simulink model "Latest_Greatest_vSandberg"  (R2022b)
settings: Solver=ode4  StartTime=0  StopTime=15  FixedStep=DeltaT  RelTol=1e-6  EnableMultiTasking=on
InitFcn:
  | %run('final_report_initexternal')
  | % Bifocal Relay Mirror Spacecraft (prior to payload installation) Dynamics Simulation          TA Sands
  | clear all;close all;clc;warning off all;
  | 
  | % Simulation run parameters
  | Rate=34.3; Rate=100;  DeltaT=1/Rate;
  | 
  | % Maneuver Parameters
  | roll=0;  pitch=0; yaw=30;   roll=roll*pi/180; pitch=pitch*pi/180; yaw=yaw*pi/180;
  | SlewStart=5; SlewTime=10; SACengage=0;
  | SlewStart=5; SlewTime=5;
  | t0=SlewTime;
  | tf=SlewTime+5;
  | %%
  | 
  | %Constants0
  | Re=6371.2e3;mu=398601.2e9;          %earth radius and universal gravitation constant
  | 
  | % tht=0.5*((sin(pi/SlewTime*(u(4)+2.5)))+1).*[u(1) u(2) u(3)]';
  | % w=(30/77.1239)*0.5*(pi/SlewTime)*((cos(pi/SlewTime*(u(4)+2.5)))+1).*[u(1) u(2) u(3)]'
  | % wdot=-(30/77.1239)*0.5*(pi/SlewTime)^(2)*((sin(pi/SlewTime*(u(4)+2.5)))).*[u(1) u(2) u(3)]'
  | 
  | %compare with differentiating in real time
  | 
  | % A0=[0 0 0];
  | % tht=A0+1/2*(1-cos(pi/SlewTime*(t-SlewStart)))*(A-A0);
  | % w=1/2*(pi/SlewTime)*sin(pi/SlewTime*(t-SlewStart))*(A-A0);
  | % wdot1=1/2*(pi/SlewTime)^2*cos(pi/SlewTime*(t-SlewStart))*(A-A0);
  | 
  | %Spacecraft orbit
  | h=0;                                     %orbit altitude
  | R=Re+h;                             %orbit radius from center of earth
  | we=0.000072921158553;   %earth's angular velocity rad/solar sec(Vallado)
  | wo=sqrt(mu/(Re+h)^3);        %orbit angular velocity
  | incln=36.6001*pi/180;          %Inclination assumed Monterey Latitude
  | epsilon=12*pi/180;  alphao=0;
  | uo=0; nuo=0;                        %Start S/C beneath subsolar point
  | betasun=60; gamma=1.5;
  | a=0.545491852; b=0.314939867;  c=0.704226952;   %Assumed spacecraft rectangular size
  | Area=[b*c a*c a*b];                 %projected area~m^2 in body x,y,z directions
  | density=4.39e-14;
  | kpre=-9.9639/24/3600/180*pi*0;      %nodal precession constant assumed zero here
  | wn=kpre*(Re/(Re+h))^3.5*cos(incln); %nodal precession (zero eccentricity)
  | V=wo*(Re+h);
  | rho=asin(Re/(h+Re));                %earth angular radius
  | Cd=2.5;     psun=4.5E-6;            %Drag coefficient and solar pressure constant~N/m^2
  | Kaero=-0.5*Cd*V^2;   Psolar=2*psun;  %constants for aero and solar torque calculation
  | dL=[0.002 0.002 0.008];             %predicted distance between cp and cg
  | Kme=2.3390e-005;
  | 
  | %Spacecraft Magnetic Properties (assumed)
  | mresid=[0 0 0.01];                  %Spacecraft residual magnetic moment
  | M=mresid;                           %Magnetic unit dipole vector
  | K=7.943e15;
  | 
  | %%
  | % Determining Principal Axes Frame
  | % ACTUAL Spacecraft Inertia conditions
  | Ix=16.67;   Iy=16.67;   Iz=16.67 ;
  | Ixy=0;  Iyz=0;  Ixz=0;
  | Imo=[Ix -Ixy -Ixz;
  |        -Ixy  Iy  -Iyz;
  |        -Ixz -Iyz  Iz];                  %Moment of inertia matrix
  | Iinv=inv(Imo);                      %Moment of inertia inverse goes in dynamics block
  | 
  | % % ACTUAL Spacecraft Inertia conditions
  | Ix=90;   Iy=100;   Iz=250 ;
  | Ixy=-10;  Iyz=20;  Ixz=-10;
  | Imo=[Ix -Ixy -Ixz;
  |        -Ixy  Iy  -Iyz;
  |        -Ixz -Iyz  Iz];                  %Moment of inertia matrix
  | Iinv=inv(Imo);                      %Moment of inertia inverse goes in dynamics block
  | 
  | [p,Ip]=eig(Imo);
  | 
  | %In this case, the principal axes line up with the body axes, otherwise we
  | %would have to examine the principal axes and see which one is closest to
  | %b1, which closest to b2, etc, to determine the order of axis to generate
  | %the DCM
  | bQp=p; %the DCM from principal axis to body are the principal axes we found
  | pQb=bQp.';
  | I1=Ip(1,1);
  | % I1=Imo(1,1);
  | I1inv=1/I1;
  | I2=Ip(2,2);
  | % I2=Imo(2,2);
  | I2inv=1/I2;
  | I3=Ip(3,3);
  | % I3=Imo(3,3);
  | I3inv=1/I3;                    %Moment of inertia inverse goes in dynamics block
  | 
  | 
  | %%
  | %FEEDFORWARD (ASSUMED) Spacecraft Inertia conditions
  | % Ix=119.1259;   Iy=150.6615;   Iz=106.0288;   %ACTUAL Values are Ix=90;   Iy=100;   Iz=250 ;
  | % Ixy=-15.7678;  Iyz=22.31637;  Ixz=-6.54859;  %ACTUAL Values are Ixy=-10;  Iyz=20;  Ixz=-10;
  | % Imo=[Ix -Ixy -Ixz;
  | %        -Ixy  Iy  -Iyz;
  | %        -Ixz -Iyz  Iz];                  %Moment of inertia matrix
  | THETAo=[Ix Ixy Ixz Iy Iyz Iz 0 0 0];
  | theta0=THETAo;
  | % theta0=[0 0 0 0 0 0 0 0 0];
  | %%
  | %Spacecraft initial Euler state angles and rates
  | phio=0;thetao=0;psio=0;                    %Initial Euler Angles
  | phidoto=0;thetadoto=0;psidoto=0;     %Initial Euler Rates
  | 
  | %Calculation of initial quaternion (qo) and angular momentum (Ho)
  | s1=sin(phio/2);s2=sin(thetao/2);s3=sin(psio/2);c1=cos(phio/2);c2=cos(thetao/2);c3=cos(psio/2);
  | q1o=s1*c2*c3-c1*s2*s3;
  | q2o=c1*s2*c3+s1*c2*s3;              %Wie pg. 321
  | q3o=c1*c2*s3-s1*s2*c3;
  | q4o=c1*c2*c3+s1*s2*s3;
  | S1=sin(phio);S2=sin(thetao);S3=sin(psio);C1=cos(phio);C2=cos(thetao);C3=cos(psio);
  | wxo=phidoto-psidoto*S2-wo*S3*C2;
  | wyo=thetadoto*C1+psidoto*C2*S1-wo*(C3*C1+S3*S2*S1);
  | wzo=psidoto*C2*C1-thetadoto*S1-wo*(S3*S2*C1-C3*S1);
  | qo=[q1o q2o q3o q4o];
  | Ho=Imo*[wxo wyo wzo]';
  | norm(Ho)*1000;
  | 
  | %Calculate eclipse time for comparison with EPS calculations
  | Te=100.87*2*V/2/pi;
  | 
  | %CMG Properties (in degrees)
  | %beta=90*pi/180;                                     %Skew angle in degrees converted to radians
  | beta=[90;90;-90;0]; beta=beta.*pi./180;
  | %beta=[54.73;54.73;-54.73;0]; beta=beta.*pi./180;
  | 
  | Gimbal0=[-30*pi/180; 90*pi/180; -30*pi/180;0];   % Initial Gimbal angles for 0 H spin up
  | w_wheel=2800*(2*pi/60);                       %Wheel speed in RPM converted to rad/s
  | Iwheel=0.0614*1.3558179483314;        % Wheel inertia in slug-ft^2 converted (exact) to kg m^2
  | h_wheel=Iwheel*w_wheel;                     % CMG Wheel Angular Momentum
  | 
  | 
  | %I believe Smeresky Rizzo did
  | %     PID_case = 1;  % Feedback controller method 1=PDI, 2=Matlab PID
  | %     kp = 1000;  % Kp gain for controller
  | %     kd = 10;  % Kd gain for controller
  | %     ki = 0.1;  % Ki gain for controller
  | %
  | %     observer_case = 2;  % 1 = observer off, 2 = observer on
  | %     kp2 = 1000;  % Kp gain for controller
  | %     kd2 = 10;  % Kd gain for controller
  | %     ki2 = 0.1;  % Ki gain for controller
  | %and used enhance PDI not just PD
  | 
  | %Smeresky Rizzo also uses
  | % J = [2.0 .1 .1; .1 2.0 .1; .1 .1 2.0]; %For an uglier J at the start time
  | % J2 = J*.2;
  | 
  | % [Fossen]'s adaptive feedforward parameters
  | ETA=1;LAMBDA=10;  uffGain=1;
  | ETA=30;
  | gamma_ff=30;
  | lambda_r=1/2; %lambda for calculation of the reference trajectories
  | lambda_r=100;
  | 
  | %FEEDBACK CONTROLLERS Follow
  | %PDI Controller Gains  % TUNED Well for Presence of LOWPASS (Kp=0.5; Kd=Kp*750;  Ki=0.1)
  | %Kp=0.5;  Kd=Kp*750;  Ki=0.1;
  | 
  | %PDI Controller Gains  % TUNED WELL FOR NO-NOISE (Kp=1; Kd=2000*Kp; Ki=5)
  | Kp=1;   Kd=Kp*6000;    Ki=5;
  | Kp=1;   Kd=1000;    Ki=1;
  | 
  | %gains for Slotine Ex 9.5
  | Kd=200;
  | Kp=Kd*lambda_r;
  | % Kp=2000;
  | 
  | %gains for Improved Hamiltonian Control
  | Kp=100;
  | Kd=200;
  | 
  | %gains for Smeresky Rizzo
  | Kp=1000*100;
  | Kd=10*100;
  | Ki=0.1*100; %added the 100 because their Inertia was about 100 times smaller
  | 
  | Ki=0;
  | 
  | %PDI Controller Gains  % TUNED WELL FOR NOISE (Kp=1; Kd=Kp*3000; Ki=1)
  | %Kp=1;   %Kd=Kp*3000;   %Ki=1;
  | 
  | %PID Controller Gains tuned well for uff and ufb decoupling
  | Kpx=1;  Kdx=1000;  Kix=-1;
  | Kpx=20;  Kdx=1000;  Kix=0.1;N_pid=100;
  | %Kpx=16.9;  Kdx=87.58;  Kix=0.8009; N_pid=5.454;
  | %Kpx=19.61;  Kdx=258.9;  Kix=0.3299; N_pid=329.6;
  | Kpx=233.9;  Kdx=890.9;  Kix=13.64; N_pid=1143;
  | Kpx=20;  Kdx=1000;  Kix=0.1;N_pid=100;
  | Kpx=100000;Kix=0.1*100;
  | %Bandpass filter pole per Bong Wie 2nd Edition pg 137-138
  | wp=10*pi/SlewTime;       % Product of pole frequency and zero frequency establishes max phase lag
  | wz=2*wp;
  | dampZ=1;  % >0 but small for good tracking..
  | dampP=dampZ;
  | % Sensor Noise Parameters
  | NoiseVariance=1e-9;             BADNoiseVariance=NoiseVariance*1e3;
  | 
  | % Observer Gains
  | MaxI=300;  lambda1=12.5  ;   lambda2=50 ;   lambda3= 200;
  | Kdo=MaxI*(lambda1+lambda2+lambda3)/10;
  | Kpo=MaxI*(lambda1*(lambda2+lambda3)+lambda2*lambda3)/10;
  | Kio=MaxI*lambda1*lambda2*lambda3/9;
  | 
  | % Kdo=1;Kpo=1;Kio=1;
  | Kdo=100;
  | Kpo=1000;
  | Kio=1000;
  | 
  | m=100*eye(3);
  | minv=pinv(m);
  | m=100;
  | x0=[R;0;0];
  | xdot0= cross([0;0;wo], x0);
  | m=100;
  | mi=1/m;
  | 
  | % Working on different parameterizations
  | % making all parameterizations the same size as the 9 parameterization,
  | % by omitting some values
  | % [u(4) 0 0 -u(2)*u(3) 0 u(3)*u(2) 0 0 0;u(1)*u(3) 0 0 u(5) 0 -u(3)*u(1) 0 0 0;-u(1)*u(2) 0 0 u(2)*u(1) 0 u(6) 0 0 0]
  | % [u(4) u(5) u(6) -u(2)*u(3) 0 u(3)*u(2) 0 0 0;u(1)*u(3) u(4) 0 u(5) u(6) -u(3)*u(1) 0 0 0;-u(1)*u(2) 0 u(4) u(2)*u(1) u(5) u(6) 0 0 0]
  | %make sure to look at what exactly theta0 is
  | 
  | 
  | 
  | % z=[u(1);u(2);u(3)]+([u(4);u(5);u(6)]-[u(1);u(2);u(3)])/2*(1+sin(pi/SlewTime*(u(8)+3*SlewTime/2-u(7))))
  | %
  | % zdot=([u(4);u(5);u(6)]-[u(1);u(2);u(3)])/2*(pi/SlewTime)*(cos(pi/SlewTime*(u(8)+3*SlewTime/2-u(7))))
  | %
  | % zddot=-([u(4);u(5);u(6)]-[u(1);u(2);u(3)])/2*(pi/SlewTime)^2*(sin(pi/SlewTime*(u(8)+3*SlewTime/2-u(7))))
  | 
  | tic
StopFcn:
  | toc
  | %run('final_report_stopexternal')
  | 
  | if flag==0; Hcmg=Hcmg;else;Hcmg=HcmgMP;end;
  | Hxcmg=[];Hycmg=[];Hzcmg=[];CondA=[]; CondA_MP=[];t=[]; SingPt=[];DetA=[];
  | for i=1:max(size(A));  t=[t i*DeltaT];  H=Hcmg(:,:,i); Hx=H(1,:);  Hy=H(2,:);  Hz=H(3,:);
  | detA=det(A(:,1:3,i));Hxcmg=[Hxcmg Hx];  Hycmg=[Hycmg Hy];  Hzcmg=[Hzcmg Hz];
  | CONDA=cond(A(:,:,i));
  | DetA=[DetA detA]; DetA=1./DetA;
  | CondA=[CondA CONDA];end;   %CondA=CondA./max(CondA); DetA=DetA./max(DetA);
  | Hmag=sqrt(Hxcmg.^2+Hycmg.^2+Hzcmg.^2);x=(max(t)-DeltaT);
  | 
  | InvCondA;
  | 
  | if flag==0; MaxInvCond=min(1./CondA(10*Rate+1:end));DELTA=delta;DELTAdot=deltadot;
  | else; MaxInvCond=min(1./CondA_MP(10*Rate+1:end));DELTA=delta_MP;DELTAdot=deltadot_MP;Hcmg=HcmgMP;end;
  | %
  | ERROR=(trajectory*180/pi-Euler);
  | 
  | figure(1); wdotTrajectory=[CMDTrajectory(:,1) CMDTrajectory(:,2) CMDTrajectory(:,3)];  wTrajectory=[CMDTrajectory(:,4) CMDTrajectory(:,5) CMDTrajectory(:,6)]; ThetaTrajectory=180/pi.*[trajectory(:,1) trajectory(:,2) trajectory(:,3)]; set(gca,'fontsize',32, 'fontname','Palatino Linotype');
  | subplot(3,1,1); plot(t,wdotTrajectory, 'linewidth',2); axis tight; grid; ylabel('\omega^d^o^t_C_M_D (deg)','fontsize',32); title('Desired Angle, Rate, Acceleration Trajectories','fontsize',32);   set(gca,'XTick',0:2:15);     set(gca,'XTickLabel',{' ',' ',' ',' ',' ',' ',' ',' ','15'}); set(gca,'fontsize',32, 'fontname','Palatino Linotype');
  | subplot(3,1,2); plot(t,wTrajectory,'linewidth',2); axis tight; grid; ylabel('\omega_C_M_D (deg)','fontsize',32);set(gca,'XTick',0:2:15);     set(gca,'XTickLabel',{' ',' ',' ',' ',' ',' ',' ',' ','15'}); set(gca,'fontsize',32, 'fontname','Palatino Linotype');
  | subplot(3,1,3); plot(t,ThetaTrajectory,'linewidth',2); axis tight; grid; ylabel('\theta_C_M_D (deg)','fontsize',32); xlabel('time (sec)','fontsize',32); set(gca,'fontsize',32, 'fontname','Palatino Linotype');
  | 
  | % figure(2);
  | % subplot(2,1,1);plot(t,Hmag,'LineWidth',3);   ylabel('|H_c_m_g|','Fontsize',16);grid;axis([0,x,0,3]); set(gca,'fontsize',16);set(gca,'XTickLabel',{' ',' ',' ',' ',' ',' ',' ',' ','15'});
  | % subplot(2,1,2);plot(t,InvCondA,'linewidth',3);grid;xlabel('t(sec)','fontsize',14,'fontname','times');ylabel('Cond[A]','fontsize',14,'fontname','times');axis([0,max(t),0,21.82]); set(gca,'fontsize',16);
  | %
  | % DELTA1=DELTA(1,:);DELTA2=DELTA(2,:);DELTA3=DELTA(3,:);DELTA4=DELTA(4,:);
  | % DELTAdot1=DELTAdot(1,:);DELTAdot2=DELTAdot(2,:);DELTAdot3=DELTAdot(3,:);DELTAdot4=DELTAdot(4,:);
  | %
  | % figure(3);subplot(4,1,1);plot(t,DELTA1,'LineWidth',3); title('Gimbal Angles','fontsize',16);ylabel('\theta_1(deg)','Fontsize',14);grid;axis tight; set(gca,'XTickLabel',{' ',' ',' ',' ',' ',' ',' ',' ','15'});set(gca,'fontsize',16);
  | % subplot(4,1,2);plot(t,DELTA2,'LineWidth',3); ylabel('\theta_2(deg)','Fontsize',16);grid;axis tight; set(gca,'XTickLabel',{' ',' ',' ',' ',' ',' ',' ',' ','15'});set(gca,'fontsize',16);
  | % subplot(4,1,3);plot(t,DELTA3,'LineWidth',3); ylabel('\theta_3(deg)','Fontsize',16);grid;axis tight; set(gca,'XTickLabel',{' ',' ',' ',' ',' ',' ',' ',' ','15'});set(gca,'fontsize',16);
  | % subplot(4,1,4);plot(t,InvCondA,'linewidth',3);grid;xlabel('t(sec)','fontsize',14,'fontname','times');ylabel('Cond[A]','fontsize',14,'fontname','times');axis([0,max(t),0,21.82]); set(gca,'fontsize',16);
  | %
  | % figure(4);subplot(4,1,1);plot(t,DELTAdot1,'LineWidth',3);  title('Gimbal Angle RATES','fontsize',16); ylabel('\theta_d_o_t_1(rad/s)','Fontsize',16);grid; axis([0,x,-pi*1.1,pi*1.1]);   set(gca,'XTickLabel',{' ',' ',' ',' ',' ',' ',' ',' ','15'});set(gca,'fontsize',16);
  | % subplot(4,1,2);plot(t,DELTAdot2,'LineWidth',3);   ylabel('\theta_d_o_t_2(rad/s)','Fontsize',16);grid;axis([0,x,-pi*1.1,pi*1.1]);   set(gca,'XTickLabel',{' ',' ',' ',' ',' ',' ',' ',' ','15'});   set(gca,'fontsize',16);
  | % subplot(4,1,3);plot(t,DELTAdot3,'LineWidth',3);   ylabel('\theta_d_o_t_3(rad/s)','Fontsize',16);grid;axis([0,x,-pi*1.1,pi*1.1]); set(gca,'XTickLabel',{' ',' ',' ',' ',' ',' ',' ',' ','15'});set(gca,'fontsize',16);
  | % subplot(4,1,4);plot(t,InvCondA,'linewidth',3);grid;xlabel('t(sec)','fontsize',14,'fontname','times');ylabel('Cond[A]','fontsize',14,'fontname','times');axis([0,max(t),0,21.82]); set(gca,'fontsize',16);
  | %
  | % figure(5);
  | % subplot(4,1,1);plot(t,Hxcmg,'linewidth',3);axis([0,x,-3.25,3.25]);grid;ylabel('h_x/|h|','fontsize',16);title('Normalized Momentum','fontsize',16);set(gca,'XTickLabel',{' ',' ',' ',' ',' ',' ',' ',' ','15'});set(gca,'fontsize',16);
  | % subplot(4,1,2);plot(t,Hycmg,'linewidth',3);axis([0,x,-3.25,3.25]);grid;ylabel('h_y/|h|','fontsize',16);set(gca,'XTickLabel',{' ',' ',' ',' ',' ',' ',' ',' ','15'});set(gca,'fontsize',16);
  | % subplot(4,1,3);plot(t,Hzcmg,'linewidth',3);axis([0,x,-3.25,3.25]);grid;ylabel('h_z/|h|','fontsize',16);  set(gca,'XTickLabel',{' ',' ',' ',' ',' ',' ',' ',' ','15'});set(gca,'fontsize',16);
  | % subplot(4,1,4);plot(t,InvCondA,'linewidth',3);grid;xlabel('t(sec)','fontsize',14,'fontname','times');ylabel('Cond[A]','fontsize',14,'fontname','times');axis([0,max(t),0,21.82]); set(gca,'fontsize',16);
  | %
  | figure(6); EulerX=Euler(:,1);EulerY=Euler(:,2);EulerZ=Euler(:,3);
  | subplot(4,1,1);plot(t,EulerX,'linewidth',3); axis([0,x,min(EulerX),max(EulerX)]);grid;ylabel('\phi(deg)','fontsize',32);title('True Euler Angles','fontsize',14);  set(gca,'XTickLabel',{' ',' ',' ',' ',' ',' ',' ',' ','15'});  set(gca,'fontsize',32, 'fontname','Palatino Linotype');
  | subplot(4,1,2);plot(t,EulerY,'linewidth',3);  axis([0,x,min(EulerY),max(EulerY)]); grid;ylabel('\theta(deg)','fontsize',32);  set(gca,'XTickLabel',{' ',' ',' ',' ',' ',' ',' ',' ','15'}); set(gca,'fontsize',32, 'fontname','Palatino Linotype');
  | subplot(4,1,3);plot(t,EulerZ,'linewidth',3);axis([0,x,min(EulerZ),max(EulerZ)]);grid;  ylabel('\psi(deg)','fontsize',32);  set(gca,'XTickLabel',{' ',' ',' ',' ',' ',' ',' ',' ','15'});  set(gca,'fontsize',32, 'fontname','Palatino Linotype');
  | subplot(4,1,4);plot(t,InvCondA,'linewidth',3);grid;xlabel('t(sec)','fontsize',32,'fontname','times');ylabel('Cond[A]','fontsize',14,'fontname','times');axis([0,max(t),0,21.82]); set(gca,'fontsize',32, 'fontname','Palatino Linotype');
  | 
  | EX=ERROR(:,1);  EY=ERROR(:,2);     EZ=ERROR(:,3);
  | MeanXerror=mean(EX); Xmean=num2str(MeanXerror); xmean=['\mu_\phi=', Xmean];
  | STDx=std(EX);Xsigma=num2str(STDx);SigmaX=['    \sigma_x=' Xsigma];  xlegend=[xmean, SigmaX];
  | MeanYerror=mean(EY); Ymean=num2str(MeanYerror); ymean=['\mu_\theta=', Ymean];
  | STDy=std(EY); Ysigma=num2str(STDy);SigmaY=['    \sigma_y=' Ysigma]; ylegend=[ymean, SigmaY];
  | MeanZerror=mean(EZ); Zmean=num2str(MeanZerror); zmean=['\mu_\psi=', Zmean];
  | STDz=std(EZ);Zsigma=num2str(STDz);SigmaZ=['    \sigma_z=' Zsigma]; zlegend=[zmean, SigmaZ];
  | MeanError=[MeanXerror MeanYerror MeanZerror];  StdDev=[STDx STDy STDz];
  | 
  | figure(7);
  | subplot(3,1,1);plot(t,EX,'linewidth',3);    axis([0,x,min(EX)*1.25,max(EX)*1.25]);  title('Euler Angle Tracking Error','fontsize',16); set(gca,'fontsize',32, 'fontname','Palatino Linotype');
  |      legend(xlegend, 'location','NorthEast');  grid   ; ylabel('\phi(deg)','fontsize',32);set(gca,'XTickLabel',{' ',' ',' ',' ',' ',' ',' ',' ','15'}); set(gca,'fontsize',32, 'fontname','Palatino Linotype');
  | subplot(3,1,2);plot(t,EY,'linewidth',3);   axis([0,x,min(EY)*1.25,max(EY)*1.25]);
  |       legend(ylegend, 'location','NorthEast');  grid;    ylabel('\theta(deg)','fontsize',32);set(gca,'XTickLabel',{' ',' ',' ',' ',' ',' ',' ',' ','15'}); set(gca,'fontsize',32, 'fontname','Palatino Linotype');
  | subplot(3,1,3);plot(t,EZ,'linewidth',3);    axis([0,x,min(EZ)*1.25,max(EZ)*1.25]);
  |      legend(zlegend, 'location','NorthEast');  grid;   ylabel('\psi(deg)','fontsize',32);xlabel('t(sec)','fontsize',16); set(gca,'fontsize',32, 'fontname','Palatino Linotype');
  | %
  | % figure(8);subplot(3,3,1);
  | % plot(t,THETAhat(:,1),'linewidth',2);grid; axis tight;ylabel('J_x_x','fontsize',16);  set(gca,'XTickLabel',{' ',' ',' ',' ',' ',' ',' ',' ','15'});  set(gca,'fontsize',16);
  | % subplot(3,3,2);plot(t,THETAhat(:,2),'linewidth',3);grid;axis tight;ylabel('J_x_y','fontsize',16);   set(gca,'XTickLabel',{' ',' ',' ',' ',' ',' ',' ',' ','15'});  set(gca,'fontsize',16);  title('Inertia & Momentum Adaption','fontsize',18);
  | % subplot(3,3,3);plot(t,THETAhat(:,3),'linewidth',3);grid;axis tight;ylabel('J_x_z','fontsize',16);set(gca,'XTickLabel',{' ',' ',' ',' ',' ',' ',' ',' ','15'});set(gca,'fontsize',16);
  | % subplot(3,3,4);plot(t,THETAhat(:,4),'linewidth',3);grid;axis tight;ylabel('J_y_y','fontsize',16);set(gca,'XTickLabel',{' ',' ',' ',' ',' ',' ',' ',' ','15'});set(gca,'fontsize',16);
  | % subplot(3,3,5);plot(t,THETAhat(:,5),'linewidth',3);grid;axis tight;ylabel('J_y_z','fontsize',16);set(gca,'XTickLabel',{' ',' ',' ',' ',' ',' ',' ',' ','15'});set(gca,'fontsize',16);
  | % subplot(3,3,6);plot(t,THETAhat(:,6),'linewidth',3);grid;axis tight;ylabel('J_z_z','fontsize',16);set(gca,'XTickLabel',{' ',' ',' ',' ',' ',' ',' ',' ','15'});set(gca,'fontsize',16);
  | % subplot(3,3,7);plot(t,THETAhat(:,7),'linewidth',3);grid;axis tight;ylabel('H_x','fontsize',16);xlabel('t(sec)','fontsize',14);set(gca,'fontsize',16);
  | % subplot(3,3,8);plot(t,THETAhat(:,8),'linewidth',3);grid;axis tight;ylabel('H_y','fontsize',16);xlabel('t(sec)','fontsize',14);set(gca,'fontsize',16);
  | % subplot(3,3,9);plot(t,THETAhat(:,9),'linewidth',3);grid;axis tight;ylabel('H_z','fontsize',16);xlabel('t(sec)','fontsize',14);set(gca,'fontsize',16);
  | %
  | ControlX=sqrt(abs(ControlEffort(end,1)))/(max(t)); ControlStringX=num2str(ControlX); Control_x=['1/t sqrt(\int u^2_\phi dt)=', ControlStringX];
  | ControlY=sqrt(abs(ControlEffort(end,2)))/(max(t)); ControlStringY=num2str(ControlY); Control_y=['1/t sqrt(\int u^2_\theta dt)=', ControlStringY];
  | ControlZ=sqrt(abs(ControlEffort(end,3)))/(max(t)); ControlStringZ=num2str(ControlZ); Control_z=['1/t sqrt(\int u^2_\psi dt)=', ControlStringZ];
  | 
  | figure(9);
  | subplot(2,1,1);plot(t,ufb,'linewidth',3);grid; axis tight;ylabel('Feedback Control (Nm)','fontname','times','fontsize',32);  legend(Control_x, Control_y, Control_z, 'location','SouthEast'); set(gca,'fontsize',32, 'fontname','Palatino Linotype');
  | title('Feedforward and Feedback Controls','fontsize',18);set(gca,'XTickLabel',{' ',' ',' ',' ',' ',' ',' ',' ','15'}); set(gca,'fontsize',32, 'fontname','Palatino Linotype');
  | subplot(2,1,2);plot(t,uff,'linewidth',3);grid; axis tight; ylabel('FeedForward Control (Nm)','fontname','times','fontsize',32);      xlabel('time(sec)','fontname','times','fontsize',14); set(gca,'fontsize',32, 'fontname','Palatino Linotype');
  | 
  | figure(10);
  | subplot(4,1,1);plot(t,ufb(:,1),'linewidth',3);grid;ylabel('u_\phi(Nm)','fontsize',32);title('u_f_b (Nm)','fontsize',32); axis tight; set(gca,'XTickLabel',{' ',' ',' ',' ',' ',' ',' ',' ','15'});set(gca,'fontsize',32, 'fontname','Palatino Linotype');
  | subplot(4,1,2);plot(t,ufb(:,2),'linewidth',3); grid;ylabel('u_\theta(Nm)','fontsize',32); axis tight; set(gca,'XTickLabel',{' ',' ',' ',' ',' ',' ',' ',' ','15'}); set(gca,'fontsize',32, 'fontname','Palatino Linotype');
  | subplot(4,1,3);plot(t,ufb(:,3),'linewidth',3); grid;ylabel('u_\psi(Nm)','fontsize',32); axis tight; set(gca,'XTickLabel',{' ',' ',' ',' ',' ',' ',' ',' ','15'}); set(gca,'fontsize',32, 'fontname','Palatino Linotype');
  | subplot(4,1,4);plot(t,InvCondA,'linewidth',3);grid;xlabel('t(sec)','fontsize',32,'fontname','times');ylabel('Cond[A]','fontsize',32,'fontname','times');axis([0,max(t),0,21.82]); set(gca,'fontsize',32, 'fontname','Palatino Linotype');
  | 
  | % % CALCULATE FIGURES OF MERIT FOR ESTIMATION ACCURACY OF LUENBERGER OBSERVER
  | % EEX=EstimationError(:,1);EEY=EstimationError(:,2);EEZ=EstimationError(:,3);
  | % MeanEEX=mean(EEX); EEXmean=num2str(MeanEEX); Exmean=['Luenberger \mu_\phi^o _E_r_r_o_r=', EEXmean];
  | % MeanEEY=mean(EEY); EEYmean=num2str(MeanEEY); Eymean=['Luenberger \mu_\theta^o _E_r_r_o_r=', EEYmean];
  | % MeanEEZ=mean(EEZ); EEZmean=num2str(MeanEEZ); Ezmean=['Luenberger \mu_\psi^o _E_r_r_o_r=', EEZmean];
  | % STDEEX=std(EEX);                      EEXstd=num2str(STDEEX);         Exstd=['   \sigma_\phi^o _E_r_r_o_r=', EEXstd];
  | % STDEEY=std(EEY);                      EEYstd=num2str(STDEEY);         Eystd=['   \sigma_\theta^o _E_r_r_o_r=', EEYstd];
  | % STDEEZ=std(EEZ);                      EEZstd=num2str(STDEEZ);         Ezstd=['   \sigma_\psi^o _E_r_r_o_r=', EEZstd];
  | % XlabelLuen=[Exmean Exstd];  YlabelLuen=[Eymean Eystd];  ZlabelLuen=[Ezmean Ezstd];
  | %
  | % % CALCULATE FIGURES OF MERIT FOR ESTIMATION ACCURACY OF PID OBSERVERS
  | % EEXo=PIDoEstimationError(:,1);EEYo=PIDoEstimationError(:,2);EEZo=PIDoEstimationError(:,3);
  | % MeanEEXo=mean(EEXo); EEXmeano=num2str(MeanEEXo); Exmeano=['PID \mu_\phi^o _E_r_r_o_r=', EEXmeano];
  | % MeanEEYo=mean(EEYo); EEYmeano=num2str(MeanEEYo); Eymeano=['PID \mu_\theta^o _E_r_r_o_r=', EEYmeano];
  | % MeanEEZo=mean(EEZo); EEZmeano=num2str(MeanEEZo); Ezmeano=['PID \mu_\psi^o _E_r_r_o_r=', EEZmeano];
  | % STDEEXo=std(EEXo);                      EEXstdo=num2str(STDEEXo);         Exstdo=['    \sigma_\phi^o _E_r_r_o_r=', EEXstdo];
  | % STDEEYo=std(EEYo);                      EEYstdo=num2str(STDEEYo);         Eystdo=['    \sigma_\theta^o _E_r_r_o_r=', EEYstdo];
  | % STDEEZo=std(EEZo);                      EEZstdo=num2str(STDEEZo);         Ezstdo=['    \sigma_\psi^o _E_r_r_o_r=', EEZstdo];
  | % XlabelPID=[Exmeano Exstdo];  YlabelPID=[Eymeano Eystdo];  ZlabelPID=[Ezmeano Ezstdo];
  | %
  | % % CALCULATE FIGURES OF MERIT FOR ESTIMATION ACCURACY OF KALMAN OBSERVERS
  | % EEXkf=KalmanEstimationError(:,1);   EEYkf=KalmanEstimationError(:,2);        EEZkf=KalmanEstimationError(:,3);
  | % MeanEEXkf=mean(EEXkf);                EEXmeankf=num2str(MeanEEXkf);         Exmeankf=['Kalman \mu_\phi^o _E_r_r_o_r=', EEXmeankf];
  | % MeanEEYkf=mean(EEYkf);                EEYmeankf=num2str(MeanEEYkf);         Eymeankf=['Kalman \mu_\theta^o _E_r_r_o_r=', EEYmeankf];
  | % MeanEEZkf=mean(EEZkf);                EEZmeankf=num2str(MeanEEZkf);         Ezmeankf=['Kalman \mu_\psi^o _E_r_r_o_r=', EEZmeankf];
  | % STDEEXkf=std(EEXkf);                      EEXstdkf=num2str(STDEEXkf);         Exstdkf=['    \sigma_\phi^o _E_r_r_o_r=', EEXstdkf];
  | % STDEEYkf=std(EEYkf);                      EEYstdkf=num2str(STDEEYkf);         Eystdkf=['    \sigma_\theta^o _E_r_r_o_r=', EEYstdkf];
  | % STDEEZkf=std(EEZkf);                      EEZstdkf=num2str(STDEEZkf);         Ezstdkf=['    \sigma_\psi^o _E_r_r_o_r=', EEZstdkf];
  | % Xlabelkf=[Exmeankf Exstdkf];  Ylabelkf=[Eymeankf Eystdkf];  Zlabelkf=[Ezmeankf Ezstdkf];
  | %
  | %figure(11);
  | %subplot(3,1,1);plot(t,KalmanEstimationError(:,1),'r:','linewidth',3); hold on; plot(t,PIDoEstimationError(:,1),'linewidth',3);  plot(t,EstimationError(:,1),'k--','linewidth',3);   set(gca,'fontsize',12);
  | %ylabel('\phi Roll (deg)','fontsize',16);   title('Observer Estimation Error Comparison','fontsize',14);  legend(Xlabelkf,XlabelPID, XlabelLuen, 'location','NorthWest'); grid; axis([0,15,-0.01,0.04]);
  | %set(gca,'XTickLabel',{' ',' ',' ',' ',' ',' ',' ',' ','15'});
  | 
  | %subplot(3,1,2); plot(t,KalmanEstimationError(:,2),'r:','linewidth',3); hold on;  plot(t,PIDoEstimationError(:,2),'linewidth',3); plot(t,EstimationError(:,2),'k--','linewidth',3); set(gca,'fontsize',12);
  | %ylabel('\theta Pitch (deg)','fontsize',16); hold off;  legend(Ylabelkf, YlabelPID, YlabelLuen, 'location','SouthWest'); grid;  set(gca,'XTickLabel',{' ',' ',' ',' ',' ',' ',' ',' ','15'});  axis([0,15,-0.08,0.03]);
  | 
  | %subplot(3,1,3); plot(t,KalmanEstimationError(:,3),'r:','linewidth',3);  hold on;  plot(t,PIDoEstimationError(:,3),'linewidth',3);plot(t,EstimationError(:,3),'k--','linewidth',3);set(gca,'fontsize',12);
  | %ylabel('\psi Yaw (deg)','fontsize',16);xlabel('t(sec)','fontsize',16);  hold off;  legend(Zlabelkf, ZlabelPID, ZlabelLuen,'location','NorthWest'); grid; axis tight;
  | 
  | %openfig('90_Degree_Singularity_Hypersurface');hold on;plot3(Hcmg(1,:),Hcmg(2,:),Hcmg(3,:), 'LineWidth',3);hold off;
  | 
  | 
  | 
  | figure(12)
  | plot(t,EX*pi/180,'linewidth',2)
  | hold on
  | plot(t,EY*pi/180,'linewidth',2)
  | plot(t,EZ*pi/180,'linewidth',2)
  | hold off
  | grid;
  | set(gca,'fontsize',32, 'fontname','Palatino Linotype');
  | %
  | % figure(13)
  | % plot(t,Euler(:,1)-30,'linewidth',2)
  | 
  | 
  | figure(13)
  | plot(t,Euler(:,1),'linewidth',2); hold on
  | plot(t,Euler(:,2),'linewidth',2); plot(t,Euler(:,3),'linewidth',2); hold off
  | cost=[' J=' num2str(sum(ControlEffort(end,:))) ';'];
  | time=[' RunTime=' num2str(toc) ';'];
  | theta_final=[' \theta(t_f)= ' num2str(Euler(end,1)) ';' cost time];
  | phi_final=[' \phi(t_f)= ' num2str(Euler(end,2)) ';'];
  | psi_final=[' \psi(t_f)= ' num2str(Euler(end,3)-30) ';'];
  | legend(theta_final,phi_final,psi_final); grid;
  | set(gca,'fontsize',32, 'fontname','Palatino Linotype');
  | 
  | % figure; grid on;
  | % plot3(r(:,1),r(:,2),r(:,3),'Linewidth',1.5);
  | %
  | % figure; grid on;
  | % plot3(r1(:,1),r1(:,2),r1(:,3),'Linewidth',1.5);
  | %
  | % plot(t,quat_error)
  | % set(gca,'fontsize',20)
undefined symbols (not defined in the file): magnitude, svd
libraries: vrlib x9, dspinverses x8, aerospace x5, matrix_library x4, simulink_need_slupdate x2, dspadpt3 x2
(part 1 of 4)
settings Model: Creator=tasands  LastModifiedBy=Cornell Gaming Lapto
settings SolverCC: AlgebraicLoopSolver=TrustRegion
settings DataIOCC: LimitDataPoints=on  SaveFormat=Array  SignalLoggingSaveFormat=ModelDataLogs  ReturnWorkspaceOutputs=off  SignalLoggingName=sigsOut
settings OptimizationCC: ExpressionDepthLimit=2147483647  InitFltsAndDblsToZero=on  LifeSpan=inf
settings DebuggingCC: SaveWithParameterizedLinksMsg=none  UnderspecifiedInitializationDetection=Classic  MergeDetectMultiDrivingBlocksExec=none  SignalResolutionControl=TryResolveAllWithWarning  MultiTaskDSMMsg=warning  MultiTaskCondExecSysMsg=none  FcnCallInpInsideContextMsg=warning  UnconnectedInputMsg=warning  UnconnectedOutputMsg=warning  UnconnectedLineMsg=warning  StateNameClashWarn=warning  PregeneratedLibrarySubsystemCodeDiagnostic=none  SFUnexpectedBacktrackingDiag=warning  SFNoUnconditionalDefaultTransitionDiag=warning  SFExecutionAtInitializationDiag=none  SFMachineParentedDataDiag=warning  ArithmeticOperatorsInVariantConditions=warning
settings HardwareCC: ProdBitPerPointer=32  ProdBitPerSizeT=32  ProdBitPerPtrDiffT=32  ProdLargestAtomicFloat=None  ProdIntDivRoundTo=Undefined  ProdEndianess=Unspecified  ProdWordSize=32  ProdHWDeviceType=32-bit Generic  TargetHWDeviceType=32-bit Generic  ProdEqTarget=off
settings ModelReferenceCC: EnableRefExpFcnMdlSchedulingChecks=on  PropagateSignalLabelsOutOfModel=off
settings SFSimCC: SimUseLocalCustomCode=off  CustomCodeUndefinedFunction=UseInterfaceOnly
settings RTWCC: RTWUseLocalCustomCode=off  DLArmComputeVersion=19.05
settings CodeAppCC: StateflowObjectComments=on
settings GRTTargetCC: TargetFcnLib=ansi_tfl_tmw.mat  TargetLangStandard=C89/C90 (ANSI)  CombineOutputUpdateFcns=off  GRTInterface=on
settings ConfigComp: CovMetricSettings=dw  CovSaveCumulativeToWorkspaceVar=on  CovSaveSingleToWorkspaceVar=on  CovExternalEMLEnable=off

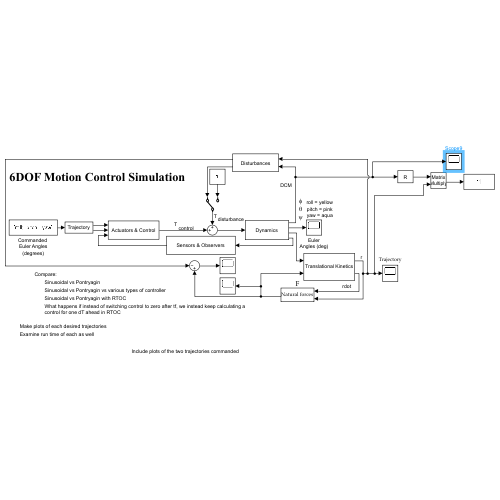
[thumbnail: Simulink's stored preview of the top-level diagram]
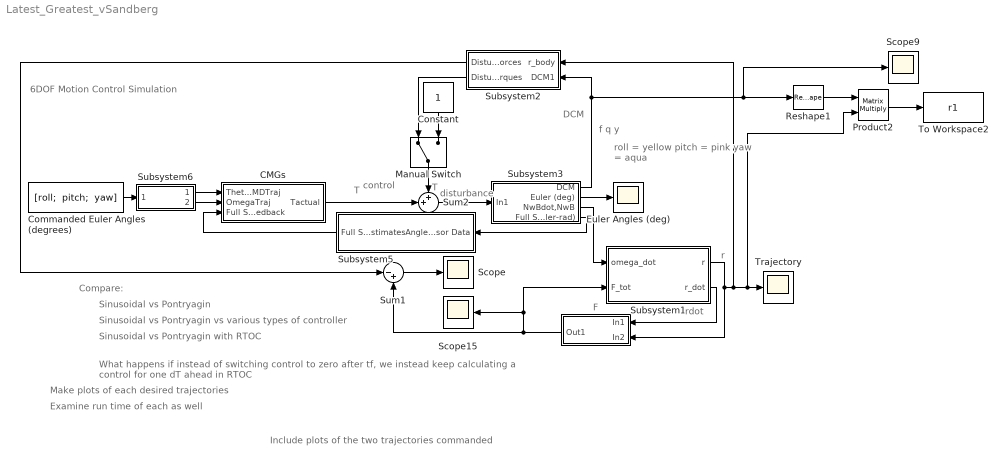
== system Latest_Greatest_vSandberg ==
  note: Include plots of the two trajectories commanded
  note: Examine run time of each as well
  note: Make plots of each desired trajectories
  note: What happens if instead of switching control to zero after tf, we instead keep calculating a control for one dT ahead in RTOC
  note: Sinusoidal vs Pontryagin with RTOC
  note: Sinusoidal vs Pontryagin vs various types of controller
  note: Sinusoidal vs Pontryagin
  note: Compare:
  note: r
  note: rdot
  note: roll = yellow
      | pitch = pink
      | yaw = aqua
  note: 6DOF Motion Control Simulation
  note: f
      | q
      | y
  note: T
  note: disturbance
  note: T
  note: control
  note: DCM
  note: F
  "     " : Subsystem
      mask Display: disp('Natural forces')
  CMGs : Subsystem
      mask Display: disp('Actuators & Control')
  "Commanded Euler Angles (degrees) " : Constant  Value="[roll;  pitch;  yaw]"
  Constant : Constant
  Euler Angles (deg) : Scope
      settings: StartFcn=|
      | %Simulink figure properties
      | shh=get(0,'ShowHiddenHandles');
      | set(0,'ShowHiddenHandles','On')
      | set(gcf,'menubar','figure')
      | set(gcf,'CloseRequestFcn','closereq')
      | set(gcf,'DefaultLineClipping','Off')
      | set(0,'ShowHiddenHandles',shh)
      | %set(gca,'LineWidth',3)
  Manual Switch : ManualSwitch
  Product2 : Product  Multiplication=Matrix(*)
  Reshape1 : Reshape  OutputDimensionality=Customize  OutputDimensions=[3,3]
  Scope : Scope
  Scope15 : Scope
  Scope9 : Scope
  Subsystem1 : Subsystem
      mask Display: disp('Translational Kinetics')
  Subsystem2 : Subsystem
      mask Display: disp('Disturbances')
  Subsystem3 : Subsystem
      mask Display: disp('Dynamics')
  Subsystem5 : Subsystem
      mask Display: disp('Sensors & Observers')
  Subsystem6 : Subsystem
      mask Display: disp('Trajectory')
  Sum1 : Sum  Inputs=|-+
  Sum2 : Sum  Inputs=++|  SaturateOnIntegerOverflow=on
  To Workspace2 : ToWorkspace  VariableName=r1  SampleTime=-1
  Trajectory : Scope
  wires:
  Sum2/1 -> Subsystem3/1(In1)
  CMGs/1(Tactual) -> Sum2/2
  Subsystem3/2(Euler (deg)) -> Euler Angles (deg)/1
  Subsystem5/1(Full State Estimates) -> CMGs/3(Full State Feedback)
  Manual Switch/1 -> Sum2/1
  Constant/1 -> Manual Switch/2
  Subsystem2/2(Disturbance Torques) -> Manual Switch/1
  Subsystem3/4(Full State Feedback  (Euler-rad)) -> Subsystem5/1(Angle & Rate Sensor Data)
  "     "/1(Out1) -> Subsystem1/2(F_tot), Scope15/1, Sum1/2
  Subsystem3/3(NwBdot,NwB) -> Subsystem1/1(omega_dot)
  Subsystem1/2(r_dot) -> "     "/1(In1)
  Sum1/1 -> Scope/1
  Product2/1 -> To Workspace2/1
  Reshape1/1 -> Product2/1
  Subsystem1/1(r) -> "     "/2(In2), Subsystem2/1(r_body), Trajectory/1, Product2/2
  Subsystem3/1(DCM) -> Subsystem2/2(DCM1), Scope9/1, Reshape1/1
  "Commanded Euler Angles (degrees) "/1 -> Subsystem6/1(Commanded Euler Angle)
  Subsystem6/1(EulerTraj) -> CMGs/1(ThetaCMDTraj)
  Subsystem6/2(EulerRateTraj) -> CMGs/2(OmegaTraj)
  Subsystem2/1(Disturbance Forces) -> Sum1/1

== system Latest_Greatest_vSandberg/      ==
  In1 : Inport
  In2 : Inport  Port=2
  " " : MATLABFcn  MATLABFcn=-0.5*Cd*density*sqrt(u(1)^2 + u(2)^2 + u(3)^2)*[u(1);u(2);u(3)]
      mask Display: disp('Drag Force')
  "  " : MATLABFcn  MATLABFcn=(-mu/(u(1)^2 + u(2)^2 + u(3)^2))*m*[u(1);u(2);u(3)]/sqrt(u(1)^2 + u(2)^2 + u(3)^2)
      mask Display: disp('Gravitational Force')
  Display : Display
  Gain : Gain
  Gain1 : Gain
  Sum1 : Sum  Inputs=|++
  Out1 : Outport
  wires:
  In1/1 -> " "/1
  In2/1 -> "  "/1
  Sum1/1 -> Out1/1
  " "/1 -> Display/1, Gain1/1
  Gain1/1 -> Sum1/2
  Gain/1 -> Sum1/1
  "  "/1 -> Gain/1

== system Latest_Greatest_vSandberg/CMGs ==
  note: TA Sands
  note: Controller & Actuators
  ThetaCMDTraj : Inport
  OmegaTraj : Inport  Port=2
  Full State Feedback : Inport  Port=3
  CMG Steering Logic1 : Subsystem
      mask Display: disp('CMG Steering & Decoupling')
  Subsystem1 : Subsystem
      mask Display: disp('displays & scopes')
  Subsystem3 : Subsystem
      mask Display: disp('Controllers')
  Tactual : Outport  VectorParamsAs1DForOutWhenUnconnected=off
  wires:
  Full State Feedback/1 -> Subsystem3/3(FullStateFeedback)
  ThetaCMDTraj/1 -> Subsystem3/1(ThetaCMDTraj)
  Subsystem3/2(u) -> CMG Steering Logic1/2(u), Subsystem1/3(In2)
  Subsystem1/1(Out1) -> Tactual/1
  CMG Steering Logic1/1(Tc) -> Subsystem1/1(In1)
  CMG Steering Logic1/2(d) -> Subsystem1/2(In3)
  Subsystem3/1(w) -> CMG Steering Logic1/1(w)
  OmegaTraj/1 -> Subsystem3/2(OmegaCMDTraj)

== system Latest_Greatest_vSandberg/Subsystem1 ==
  note: $^B\dot r$
  note: $r$
  note: $^I\ddot r=^B\ddot r+^B\dot\omega \times r+2\omega\times ^B\dot r+\omega\times(\omega\times r)$
  note: Where $^B\ddot r$ is the acceleration in the body frame and the other terms are the Euler Force, the Coriolis Force, and the Centripetal Force
  note: We can also say, that the acceleration relative to the body frame, expressed in the body frame is...
  note: The "real" forces minus the "imaginary" forces, the Euler, Coriolis, and Cetripetal forces.
  note: As the "real" forces are what define the acceleration relative to the INERTIAL frame by application of Newtons law
  note: $^B\ddot r=F/m-[^B\dot\omega\times r +2\omega\times^B\dot r+ \omega\times(\omega\times r)]$
  note: $F_{tot}$
  note: $^B\dot\omega$
  note: $\omega$
  note: $F/m$
  note: Euler Force
  note: Centripetal Force
  note: Coriolis Force
  omega_dot : Inport
  F_tot : Inport  Port=2
  Cross Product{,1..3} (4 alike) : vrlib/Utilities/Cross Product
  Demux : Demux  Outputs=2
  Gain : Gain  Gain=2
  Gain1 : Gain
  Gain2 : Gain
  Gain3 : Gain
  Gain4 : Gain  Gain=mi
  Integrator : Integrator  InitialCondition=xdot0
  Integrator1 : Integrator  InitialCondition=x0
  Scope : Scope
  Sum : Sum  Inputs=|+-
  Sum1 : Sum  Inputs=|++
  Sum2 : Sum  Inputs=|++
  To Workspace2 : ToWorkspace  VariableName=r  SampleTime=-1
  r : Outport
  r_dot : Outport  Port=2
  wires:
  F_tot/1 -> Gain4/1
  Demux/1 -> Cross Product/1
  omega_dot/1 -> Demux/1
  Integrator1/1 -> Cross Product/2, Cross Product1/2, To Workspace2/1, r/1
  Integrator/1 -> r_dot/1, Cross Product3/2, Integrator1/1
  Sum1/1 -> Sum2/2
  Cross Product/1 -> Gain1/1
  Gain/1 -> Gain2/1
  Cross Product2/1 -> Gain3/1
  Cross Product3/1 -> Gain/1
  Cross Product1/1 -> Cross Product2/2
  Demux/2 -> Cross Product2/1, Cross Product3/1, Cross Product1/1
  Sum2/1 -> Sum/2
  Gain1/1 -> Sum2/1
  Gain2/1 -> Sum1/2
  Gain3/1 -> Sum1/1
  Sum/1 -> Integrator/1
  Gain4/1 -> Scope/1, Sum/1

== system Latest_Greatest_vSandberg/Subsystem2 ==
  r_body : Inport
  DCM1 : Inport  Port=2
  Subsystem : Subsystem  Commented=on
  Subsystem1 : Subsystem
  Sum1 : Sum  Commented=on  Inputs=+++  SaturateOnIntegerOverflow=on
  Sum2 : Sum  Inputs=+++  SaturateOnIntegerOverflow=on
  Sum3 : Sum  SaturateOnIntegerOverflow=on
  Disturbance Forces : Outport
  Disturbance Torques : Outport  Port=2
  wires:
  Subsystem/1(Magnetic Disturbance) -> Sum1/1
  Subsystem/3(Gravity Gradient Disturbance) -> Sum1/3
  Sum1/1 -> ?
  Subsystem/2(Aero & Solar Disturbances) -> Sum1/2
  Subsystem1/4(Aero & Solar Disturbance Forces) -> Sum3/1
  Sum2/1 -> Disturbance Torques/1
  DCM1/1 -> Subsystem1/1(DCM)
  Subsystem1/1(Magnetic Disturbance) -> Sum2/1
  Subsystem1/3(Gravity Gradient Disturbance) -> Sum2/3
  r_body/1 -> Subsystem1/2(r_body)
  Sum3/1 -> Disturbance Forces/1
  Subsystem1/2(Aero & Solar Disturbances) -> Sum2/2
  Subsystem1/5(Gravity Gradient Disturbance Force) -> Sum3/2

== system Latest_Greatest_vSandberg/Subsystem3 ==
  note: w
  note: N B
  note: N B
  In1 : Inport
  Body Dynamics : Subsystem
      mask Display: disp('TASS2 Dynamics')
  Euler RATES (deg/s) : Scope
      settings: StopFcn=|
      | %Simulink figure properties
      | shh=get(0,'ShowHiddenHandles');
      | set(0,'ShowHiddenHandles','On')
      | set(gcf,'menubar','figure')
      | set(gcf,'CloseRequestFcn','closereq')
      | set(gcf,'DefaultLineClipping','Off')
      | set(0,'ShowHiddenHandles',shh)
  Mux : Mux  Inputs=2
  Mux1 : Mux  Inputs=2
  Subsystem1 : Subsystem
      mask Display: disp('Kinematics')
  DCM : Outport  VectorParamsAs1DForOutWhenUnconnected=off
  Euler (deg) : Outport  Port=2  VectorParamsAs1DForOutWhenUnconnected=off
  NwBdot,NwB : Outport  Port=3
  Full State Feedback  (Euler-rad) : Outport  Port=4  VectorParamsAs1DForOutWhenUnconnected=off
  tag scope: ActualEuler=global
  wires:
  Subsystem1/1(DCM) -> DCM/1
  In1/1 -> Body Dynamics/1(T)
  Subsystem1/2(Euler(deg)) -> Euler (deg)/1, [ActualEuler]
  Subsystem1/3(Euler(rad)) -> Mux/1
  Mux/1 -> Full State Feedback  (Euler-rad)/1
  Mux1/1 -> NwBdot,NwB/1
  Body Dynamics/1(NwB) -> Subsystem1/1(wbn), Mux1/2, Mux/2, Euler RATES (deg/s)/1
  Body Dynamics/2(NwBdot) -> Mux1/1

== system Latest_Greatest_vSandberg/Subsystem5 ==
  note: FULL STATE FEEDBACK (IDEAL)
  note: FULL STATE FEEDBACK (SENSOR)
  Angle & Rate Sensor Data : Inport
  Manual Switch : ManualSwitch
  Manual Switch1 : ManualSwitch  CurrentSetting=0
  Manual Switch2 : ManualSwitch  CurrentSetting=0
  Manual Switch3 : ManualSwitch
  Manual Switch4 : ManualSwitch
  OBSERVERS (MASK THIS SUBSYSTEM AS CLASS DEMO)1 : Subsystem
      mask Display: disp('Observer')
  Subsystem2 : Subsystem
      mask Display: disp('Sensor')
  Subsystem4 : Subsystem
      mask Display: disp('Kalman Filter')
  Subsystem5 : Subsystem
      mask Display: disp('Lowpass Filter')
  Full State Estimates : Outport  VectorParamsAs1DForOutWhenUnconnected=off
  wires:
  Angle & Rate Sensor Data/1 -> Manual Switch3/1, Subsystem2/1(Full State Feedback)
  Subsystem4/1(Out1) -> Manual Switch1/1
  Manual Switch1/1 -> Manual Switch/2
  Manual Switch2/1 -> Subsystem4/1(Full State Feedback)
  OBSERVERS (MASK THIS SUBSYSTEM AS CLASS DEMO)1/1(Estimated full state feedback (Euler-rad)) -> Manual Switch1/2, Manual Switch2/2
  Manual Switch3/1 -> Manual Switch/1
  Manual Switch4/1 -> Full State Estimates/1
  Manual Switch/1 -> Manual Switch4/1, Subsystem5/1(u)
  Subsystem2/1(Noisy State Feedback) -> Manual Switch2/1, Manual Switch3/2, OBSERVERS (MASK THIS SUBSYSTEM AS CLASS DEMO)1/1(Full State Feedback)
  Subsystem5/1(u(filtered)) -> Manual Switch4/2

== system Latest_Greatest_vSandberg/Subsystem6 ==
  Commanded Euler Angle : Inport
  "   " : Mux  Inputs=3
  Demux : Demux  Outputs=3
  Manual Switch1 : ManualSwitch  CurrentSetting=0
  Manual Switch2 : ManualSwitch
  Mux1 : Mux  Inputs=3
  Mux4 : Mux  Inputs=3
  Subsystem1 : Subsystem
      mask Display: disp('Versine Slew')
  Subsystem2 : Subsystem
      mask Display: disp('To Workspace')
  Subsystem3 : Subsystem
      mask Display: disp('Pontryagin Optimal Trajectory \n Non-principal Frame')
  Subsystem6 : Subsystem
      mask Display: disp('Pontryagin Optimal Trajectory')
  To Workspace : ToWorkspace  VariableName=trajectory  SampleTime=-1
  EulerTraj : Outport
  EulerRateTraj : Outport  Port=2
  tag scope: OmegaDotTrajectory=global
  wires:
  Demux/2 -> EulerRateTraj/1
  Subsystem1/1(EulerAngleTraj) -> Mux1/1
  Subsystem1/2(EulerRateTraj) -> Mux1/2
  Subsystem1/3(OmegaDotTrajectory) -> Mux1/3
  Commanded Euler Angle/1 -> Subsystem3/1(Commanded Euler Angle), Subsystem6/1(Commanded Euler Angle), Subsystem2/1(In1), Subsystem1/1(Commanded Euler Angle)
  Demux/3 -> [OmegaDotTrajectory]
  Subsystem6/1(EulerAngleTraj) -> Mux4/1
  Subsystem6/2(EulerRateTraj) -> Mux4/2
  Subsystem6/3(OmegaDotTraj1) -> Mux4/3
  Mux4/1 -> Manual Switch2/2
  Mux1/1 -> Manual Switch2/1
  Subsystem3/1(EulerAngleTraj) -> "   "/1
  Subsystem3/2(EulerRateTraj) -> "   "/2
  Subsystem3/3(OmegaDotTraj1) -> "   "/3
  Manual Switch2/1 -> Manual Switch1/1
  "   "/1 -> Manual Switch1/2
  Manual Switch1/1 -> Demux/1
  Demux/1 -> To Workspace/1, EulerTraj/1

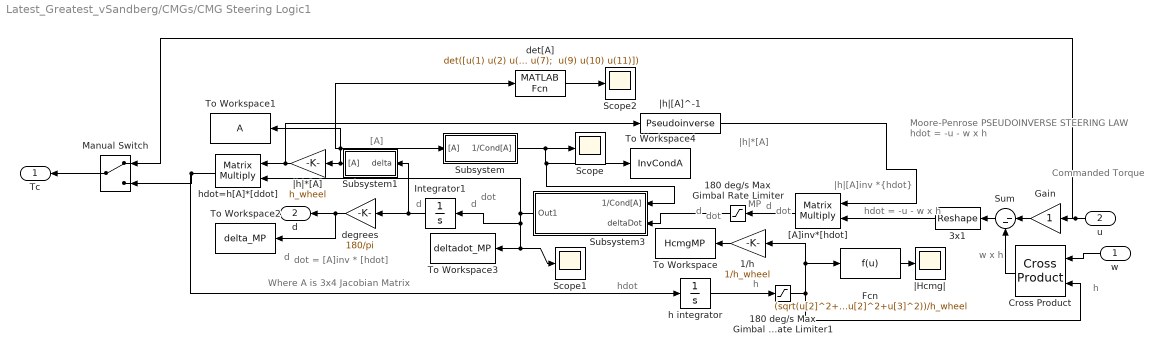
== system Latest_Greatest_vSandberg/CMGs/CMG Steering Logic1 ==
  note: MP
  note: d
  note: dot
  note: d
  note: [A]
  note: |h|*[A]
  note: h
  note: dot
  note: d
  note: |h|[A]inv *{hdot}
  note: Commanded
      | Torque
  note: Where A is 3x4 Jacobian Matrix
  note: d
  note: dot = [A]inv * [hdot]
  note: Moore-Penrose
      | PSEUDOINVERSE STEERING LAW
      | hdot = -u - w x h
  note: w x h
  note: dot
  note: d
  note: hdot = -u - w x h
  note: h
  note: hdot
  w : Inport
  u : Inport  Port=2
  1/h : Gain  Gain=1/h_wheel
  180 deg/s Max Gimbal Rate Limiter : Saturate  UpperLimit=pi  LowerLimit=-pi
  180 deg/s Max Gimbal Rate Limiter1 : Saturate  UpperLimit=[h_wheel;2*h_wheel;3*h_wheel]  LowerLimit=-1
  3x1 : Reshape  OutputDimensionality=Customize  OutputDimensions=[3,1]
  Cross Product : matrix_library/Cross Product
  Fcn : Fcn  Expr=(sqrt(u[2]^2+u[2]^2+u[3]^2))/h_wheel
  Gain : Gain
  Integrator1 : Integrator  InitialCondition=Gimbal0
  Manual Switch : ManualSwitch
  Scope : Scope
  Scope1 : Scope
  Scope2 : Scope
  Subsystem : Subsystem
      mask Display: disp('1/Cond[A]')
  Subsystem1 : Subsystem
      mask Display: disp('[A] Matrix')
  Subsystem3 : Subsystem
      mask Display: disp('SPUD')
  Sum : Sum  Inputs=|--  SaturateOnIntegerOverflow=on
  To Workspace : ToWorkspace  VariableName=HcmgMP  SampleTime=-1
  To Workspace1 : ToWorkspace  VariableName=A  SampleTime=-1
  To Workspace2 : ToWorkspace  VariableName=delta_MP  SampleTime=-1
  To Workspace3 : ToWorkspace  VariableName=deltadot_MP  SampleTime=-1
  To Workspace4 : ToWorkspace  VariableName=InvCondA  SampleTime=-1
  "[A]inv*[hdot]" : Product  Multiplication=Matrix(*)  SaturateOnIntegerOverflow=on  OutDataTypeStr=Inherit: Same as first input
  degrees : Gain  Gain=180/pi
  det[A] : MATLABFcn  MATLABFcn="det([u(1) u(2) u(3);  u(5) u(6) u(7);  u(9) u(10) u(11)])"
  h integrator : Integrator
  hdot=h[A]*[ddot] : Product  Multiplication=Matrix(*)  SaturateOnIntegerOverflow=on  OutDataTypeStr=Inherit: Same as first input
  |Hcmg| : Scope
  |h|*[A] : Gain  Gain=h_wheel
  |h|[A]^-1 : dspinverses/Pseudoinverse  wanterr=off  SimulateUsing=Interpreted execution
  Tc : Outport  VectorParamsAs1DForOutWhenUnconnected=off
  d : Outport  Port=2  VectorParamsAs1DForOutWhenUnconnected=off
  wires:
  Subsystem3/1(Out1) -> Integrator1/1, To Workspace3/1, Scope1/1, hdot=h[A]*[ddot]/2
  180 deg/s Max Gimbal Rate Limiter/1 -> Subsystem3/2(deltaDot)
  degrees/1 -> To Workspace2/1, d/1
  Integrator1/1 -> degrees/1, Subsystem1/1(delta)
  Subsystem1/1("[A]") -> det[A]/1, To Workspace1/1, Subsystem/1("[A]"), |h|*[A]/1
  Fcn/1 -> |Hcmg|/1
  "[A]inv*[hdot]"/1 -> 180 deg/s Max Gimbal Rate Limiter/1
  180 deg/s Max Gimbal Rate Limiter1/1 -> Cross Product/2, 1/h/1, Fcn/1
  3x1/1 -> "[A]inv*[hdot]"/2
  |h|*[A]/1 -> |h|[A]^-1/1, hdot=h[A]*[ddot]/1
  hdot=h[A]*[ddot]/1 -> Manual Switch/2, h integrator/1
  u/1 -> Manual Switch/1, Gain/1
  Sum/1 -> 3x1/1
  w/1 -> Cross Product/1
  Cross Product/1 -> Sum/2
  h integrator/1 -> 180 deg/s Max Gimbal Rate Limiter1/1
  1/h/1 -> To Workspace/1
  det[A]/1 -> Scope2/1
  |h|[A]^-1/1 -> "[A]inv*[hdot]"/1
  Subsystem/1(1/Cond[A]) -> Scope/1, Subsystem3/1(1/Cond[A]), To Workspace4/1
  Manual Switch/1 -> Tc/1
  Gain/1 -> Sum/1

== system Latest_Greatest_vSandberg/CMGs/Subsystem1 ==
  In1 : Inport
  In3 : Inport  Port=2
  In2 : Inport  Port=3
  Displays : Subsystem
      mask Display: disp('Displays')
  Subsystem : Subsystem
      mask Display: disp('DeMux')
  Subsystem2 : Subsystem
      mask Display: disp('CMGs')
  Out1 : Outport  VectorParamsAs1DForOutWhenUnconnected=off
  wires:
  Subsystem/1(Torque) -> Displays/1(Tc), Out1/1
  Subsystem/2(GimbalAngles) -> Displays/2(d)
  In2/1 -> Displays/3(u)
  Subsystem2/1(MP) -> Subsystem/1(SAC/MP)
  In1/1 -> Subsystem2/1(u)
  In3/1 -> Subsystem2/2(gimbal angles)

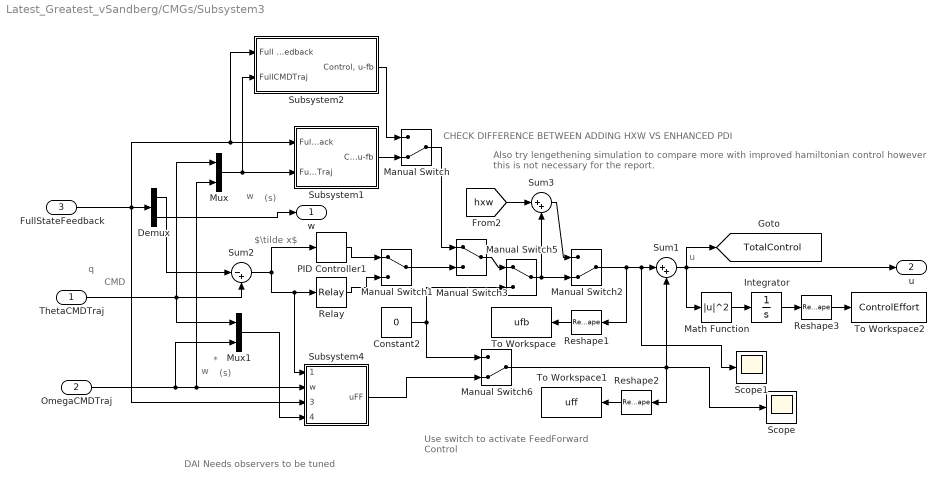
== system Latest_Greatest_vSandberg/CMGs/Subsystem3 ==
  note: Also try lengethening simulation to compare more with improved hamiltonian control however this is not necessary for the report.
  note: CHECK DIFFERENCE BETWEEN ADDING HXW VS ENHANCED PDI
  note: DAI Needs observers to be tuned
  note: u
  note: $\tilde x$
  note: Use switch to activate
      | FeedForward Control
  note: w
  note: (s)
  note: q
  note: CMD
  note: *
  note: (s)
  note: w
  ThetaCMDTraj : Inport
  OmegaCMDTraj : Inport  Port=2
  FullStateFeedback : Inport  Port=3
  Constant2 : Constant  Value=0
  Demux : Demux  Outputs=2
  Integrator : Integrator
  Manual Switch : ManualSwitch  CurrentSetting=0
  Manual Switch1 : ManualSwitch
  Manual Switch2 : ManualSwitch  CurrentSetting=0
  Manual Switch3 : ManualSwitch
  Manual Switch5 : ManualSwitch
  Manual Switch6 : ManualSwitch  CurrentSetting=0
  Math Function : Math  Operator=magnitude^2  SignedPower=on
  Mux : Mux  Inputs=2
  Mux1 : Mux  Inputs=2
  PID Controller1 : simulink_need_slupdate/PID Controller  P=Kpx  I=0  D=Kdx
  Relay : Relay  OnOutputValue=pi  OffOutputValue=-pi
  Reshape1 : Reshape  OutputDimensions=[1,9]
  Reshape2 : Reshape  OutputDimensions=[1,9]
  Reshape3 : Reshape  OutputDimensions=[1,9]
  Scope : Scope
  Scope1 : Scope
  Subsystem1 : Subsystem
      mask Display: disp('PDI Controller')
  Subsystem2 : Subsystem
      mask Display: disp('Enhanced PDI Controller')
  Subsystem4 : Subsystem
      mask Display: disp('Feedforward')
  Sum1 : Sum  Inputs=|++  SaturateOnIntegerOverflow=on
  Sum2 : Sum  Inputs=|-+  SaturateOnIntegerOverflow=on
  Sum3 : Sum  Inputs=|++  SaturateOnIntegerOverflow=on
  To Workspace : ToWorkspace  VariableName=ufb  SampleTime=-1
  To Workspace1 : ToWorkspace  VariableName=uff  SampleTime=-1
  To Workspace2 : ToWorkspace  VariableName=ControlEffort  SampleTime=-1
  w : Outport  VectorParamsAs1DForOutWhenUnconnected=off
  u : Outport  Port=2  VectorParamsAs1DForOutWhenUnconnected=off
  tag scope: TotalControl=global
  wires:
  Demux/1 -> Sum2/1
  ThetaCMDTraj/1 -> Mux1/1, Sum2/2, Mux/1
  Relay/1 -> Manual Switch1/2
  PID Controller1/1 -> Manual Switch1/1
  Manual Switch1/1 -> Manual Switch3/2
  Demux/2 -> w/1
  Subsystem1/1("Control, u-fb") -> Manual Switch/2
  FullStateFeedback/1 -> Subsystem1/1(Full State Feedback), Subsystem2/1(Full State Feedback), Demux/1, Subsystem4/3(State Feedback)
  Sum1/1 -> [TotalControl], u/1, Math Function/1
  Math Function/1 -> Integrator/1
  Integrator/1 -> Reshape3/1
  Reshape1/1 -> To Workspace/1
  Reshape2/1 -> To Workspace1/1
  Reshape3/1 -> To Workspace2/1
  Manual Switch3/1 -> Manual Switch5/1
  Manual Switch6/1 -> Scope/1, Sum1/2, Reshape2/1
  Constant2/1 -> Manual Switch5/2, Manual Switch6/1
  Subsystem4/1(uFF) -> Manual Switch6/2
  Manual Switch5/1 -> Manual Switch2/2, Sum3/2
  Manual Switch2/1 -> Scope1/1, Sum1/1, Reshape1/1
  Sum3/1 -> Manual Switch2/1
  [hxw] -> Sum3/1
  OmegaCMDTraj/1 -> Mux1/2, Subsystem4/2(w), Mux/2
  Mux/1 -> Subsystem1/2(FullCMDTraj), Subsystem2/2(FullCMDTraj)
  Sum2/1 -> Subsystem4/1(LAMBDA*xtilda), Relay/1, PID Controller1/1
  Mux1/1 -> Subsystem4/4(Trajectory Desired)
  Subsystem2/1("Control, u-fb") -> Manual Switch/1
  Manual Switch/1 -> Manual Switch3/1

== system Latest_Greatest_vSandberg/Subsystem2/Subsystem ==
  note: DCM
  note: DCM
  DCM : Inport
  Gravity Gradient : Subsystem
  Magnetic Torque : Subsystem
  On/Off : Gain  Gain=0  SaturateOnIntegerOverflow=on  OutDataTypeStr=Inherit: Same as input  ParamDataTypeStr=Inherit: Same as input
  "On/Off " : Gain  SaturateOnIntegerOverflow=on  OutDataTypeStr=Inherit: Same as input  ParamDataTypeStr=Inherit: Same as input
  On/off : Gain  Gain=0  SaturateOnIntegerOverflow=on  OutDataTypeStr=Inherit: Same as input  ParamDataTypeStr=Inherit: Same as input
  Orbit parameters : Subsystem
  TAero & Tsolar : Subsystem
  Magnetic Disturbance : Outport
  Aero & Solar Disturbances : Outport  Port=2
  Gravity Gradient Disturbance : Outport  Port=3
  wires:
  Gravity Gradient/1(Tgg) -> "On/Off "/1
  TAero & Tsolar/1(Taero & Tsolar) -> On/off/1
  Orbit parameters/4(nu) -> TAero & Tsolar/1(nu)
  Orbit parameters/1(alpha) -> Magnetic Torque/2(alpha)
  Orbit parameters/2(incln) -> Magnetic Torque/3(inclination)
  Orbit parameters/3(u) -> Magnetic Torque/4(u)
  Magnetic Torque/1(Sb) -> On/Off/1
  DCM/1 -> Magnetic Torque/1(DCM), TAero & Tsolar/2(DCM), Gravity Gradient/1(DCM)
  On/Off/1 -> Magnetic Disturbance/1
  On/off/1 -> Aero & Solar Disturbances/1
  "On/Off "/1 -> Gravity Gradient Disturbance/1
